simulink model "NumericalExampleWithSolids"  (R2024b)
settings: Solver=VariableStepDiscrete  StartTime=0.0  StopTime=T_final  MaxStep=0.4  MinStep=0.5  RelTol=1e-3
values from neighbouring files (symbols this model uses):
  loss_due_to_contamination = 0.3    [NumericalExampleWithSolids_param.m]
  m_ini_2_HDPE = 20    [NumericalExampleWithSolids_param.m]
  m_ini_2_PET = 20    [NumericalExampleWithSolids_param.m]
  m_ini_2_PP = 20    [NumericalExampleWithSolids_param.m]
  m_ini_3_HDPE = 100    [NumericalExampleWithSolids_param.m]
  m_ini_3_PET = 150    [NumericalExampleWithSolids_param.m]
  m_ini_3_PP = 120    [NumericalExampleWithSolids_param.m]
  m_ini_HDPE = 4.1    [NumericalExampleWithSolids_param.m]
  m_ini_PET = 8.1    [NumericalExampleWithSolids_param.m]
  m_ini_PP = 4.4    [NumericalExampleWithSolids_param.m]
  m_ini_Transport1to2_HDPE = 0    [NumericalExampleWithSolids_param.m]
  m_ini_Transport1to2_PET = 0    [NumericalExampleWithSolids_param.m]
  m_ini_Transport1to2_PP = 0    [NumericalExampleWithSolids_param.m]
  m_ini_Transport2to1_HDPE = 0    [NumericalExampleWithSolids_param.m]
  m_ini_Transport2to1_PET = 0    [NumericalExampleWithSolids_param.m]
  m_ini_Transport2to1_PP = 0    [NumericalExampleWithSolids_param.m]
  m_ini_Transport3to1_HDPE = 0    [NumericalExampleWithSolids_param.m]
  m_ini_Transport3to1_PET = 0    [NumericalExampleWithSolids_param.m]
  m_ini_Transport3to1_PP = 0    [NumericalExampleWithSolids_param.m]
  m_out_3_HDPE = 0.5    [NumericalExampleWithSolids_param.m]
  m_out_3_PET = 2    [NumericalExampleWithSolids_param.m]
  m_out_3_PP = 1    [NumericalExampleWithSolids_param.m]
  m_out_HDPE = 4.1    [NumericalExampleWithSolids_param.m]
  m_out_PET = 8.1    [NumericalExampleWithSolids_param.m]
  m_out_PP = 4.4    [NumericalExampleWithSolids_param.m]
  t_out_2_HDPE = t_out_Transport1to2_HDPE + recycling_time    (= 260)    [NumericalExampleWithSolids_param.m]
  t_out_2_PET = t_out_Transport1to2_PET + recycling_time    (= 260)    [NumericalExampleWithSolids_param.m]
  t_out_2_PP = t_out_Transport1to2_PP + recycling_time    (= 260)    [NumericalExampleWithSolids_param.m]
  t_out_3_HDPE = 1    [NumericalExampleWithSolids_param.m]
  t_out_3_PET = 1    [NumericalExampleWithSolids_param.m]
  t_out_3_PP = 1    [NumericalExampleWithSolids_param.m]
  t_out_HDPE = 100    [NumericalExampleWithSolids_param.m]
  t_out_PET = 100    [NumericalExampleWithSolids_param.m]
  t_out_PP = 100    [NumericalExampleWithSolids_param.m]
  t_out_Transport1to2_HDPE = t_out_HDPE + transportation_time_1to2    (= 220)    [NumericalExampleWithSolids_param.m]
  t_out_Transport1to2_PET = t_out_PET + transportation_time_1to2    (= 220)    [NumericalExampleWithSolids_param.m]
  t_out_Transport1to2_PP = t_out_PP + transportation_time_1to2    (= 220)    [NumericalExampleWithSolids_param.m]
  t_out_Transport2to1_HDPE = t_out_2_HDPE + transportation_time_2to1    (= 290)    [NumericalExampleWithSolids_param.m]
  t_out_Transport2to1_PET = t_out_2_PET + transportation_time_2to1    (= 290)    [NumericalExampleWithSolids_param.m]
  t_out_Transport2to1_PP = t_out_2_PP + transportation_time_2to1    (= 290)    [NumericalExampleWithSolids_param.m]
  t_out_Transport3to1_HDPE = t_out_3_HDPE + transportation_time_3to1    (= 7)    [NumericalExampleWithSolids_param.m]
  t_out_Transport3to1_PET = t_out_3_PET + transportation_time_3to1    (= 7)    [NumericalExampleWithSolids_param.m]
  t_out_Transport3to1_PP = t_out_3_PP + transportation_time_3to1    (= 7)    [NumericalExampleWithSolids_param.m]
  transportation_time_1to2 = 60*hours_for_transportation_1to2    (= 120)    [NumericalExampleWithSolids_param.m]
  transportation_time_2to1 = 60*hours_for_transportation_2to1    (= 30)    [NumericalExampleWithSolids_param.m]
  transportation_time_3to1 = 60*hours_for_transportation_3to1    (= 6)    [NumericalExampleWithSolids_param.m]
libraries: dspstat3 x1

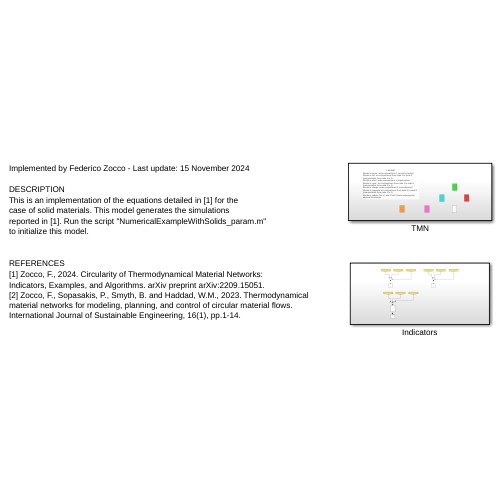
[thumbnail: Simulink's stored preview of the top-level diagram]
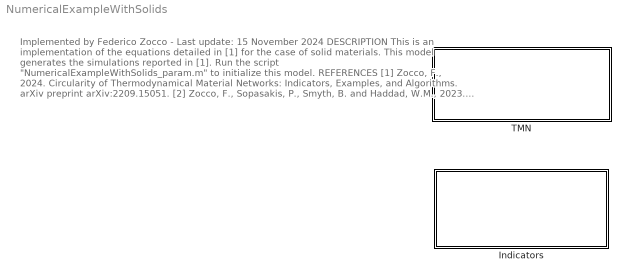
== system NumericalExampleWithSolids ==
  note: Implemented by Federico Zocco - Last update: 15 November 2024
      |
      | DESCRIPTION
      | This is an implementation of the equations detailed in [1] for the
      | case of solid materials. This model generates the simulations
      | reported in [1]. Run the script "NumericalExampleWithSolids_param.m"
      | to initialize this model.
      |
      | REFERENCES
      | [1] Zocco, F., 2024. Circularity of Thermodynamical Material Networks:
      | Indicators, Examples, and Algorithms. arXiv preprint arXiv:2209.15051.
      | [2] Zocco, F., Sopasakis, P., Smyth, B. and Haddad, W.M., 2023. Thermodynamical material networks for modeling, planning, and control of circular material flows. International Journal of Sustainable Engineering, 16(1), pp.1-14.
  Indicators : Subsystem
  TMN : Subsystem

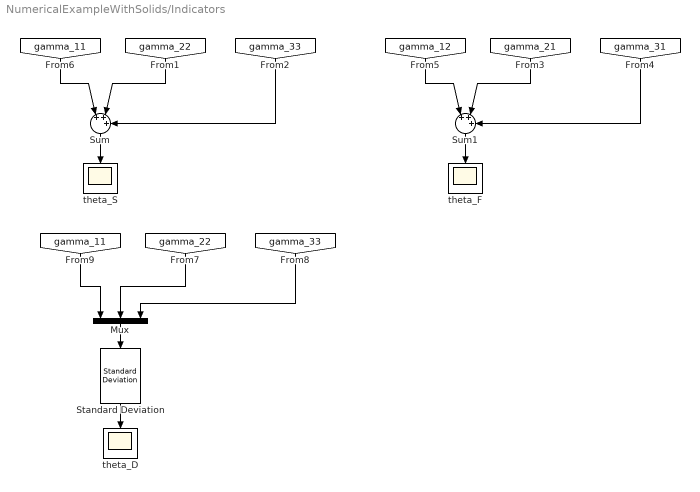
== system NumericalExampleWithSolids/Indicators ==
  Mux : Mux  Inputs=3
  Standard Deviation : dspstat3/Standard Deviation  run=off  directionMode=Each column  dimension=1  InputProcessing=Columns as channels (frame based)  reset_popup=None  roiEnable=off  roiType=Rectangles  roiPortion=Entire ROI  roiOutput=Individual statistics for each ROI  roiFlag=off
  Sum : Sum  Inputs=|+++
  Sum1 : Sum  Inputs=|+++
  theta_D : Scope
  theta_F : Scope
  theta_S : Scope
  wires:
  Mux/1 -> Standard Deviation/1
  [gamma_12] -> Sum1/1
  [gamma_22] -> Mux/2
  Sum/1 -> theta_S/1
  [gamma_33] -> Mux/3
  Standard Deviation/1 -> theta_D/1
  [gamma_11] -> Sum/1
  [gamma_33] -> Sum/3
  [gamma_31] -> Sum1/3
  Sum1/1 -> theta_F/1
  [gamma_21] -> Sum1/2
  [gamma_22] -> Sum/2
  [gamma_11] -> Mux/1

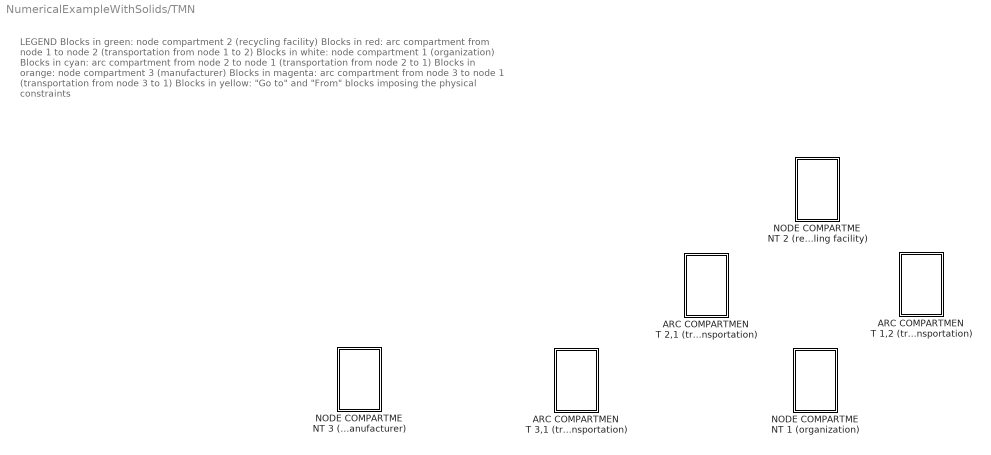
== system NumericalExampleWithSolids/TMN ==
  note: LEGEND
      | Blocks in green: node compartment 2 (recycling facility)
      | Blocks in red: arc compartment from node 1 to node 2 (transportation from node 1 to 2)
      | Blocks in white: node compartment 1 (organization)
      | Blocks in cyan: arc compartment from node 2 to node 1 (transportation from node 2 to 1)
      | Blocks in orange: node compartment 3 (manufacturer)
      | Blocks in magenta: arc compartment from node 3 to node 1 (transportation from node 3 to 1)
      | Blocks in yellow: "Go to" and "From" blocks imposing the physical constraints
  ARC COMPARTMENT 1,2 (transportation) : Subsystem
  ARC COMPARTMENT 2,1 (transportation) : Subsystem
  ARC COMPARTMENT 3,1 (transportation) : Subsystem
  NODE COMPARTMENT 1 (organization) : Subsystem
  NODE COMPARTMENT 2 (recycling facility) : Subsystem
  NODE COMPARTMENT 3 (manufacturer) : Subsystem

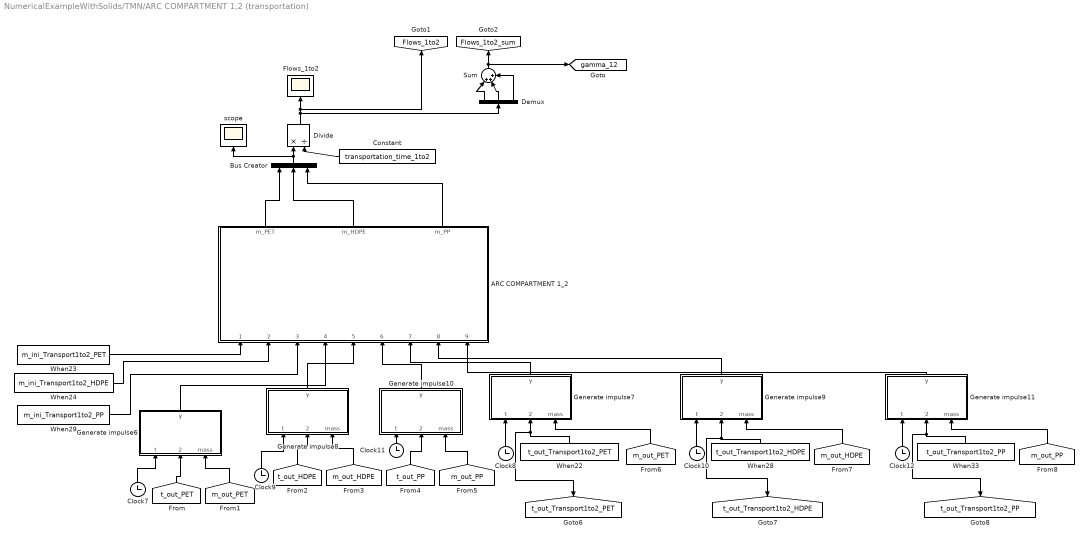
== system NumericalExampleWithSolids/TMN/ARC COMPARTMENT 1,2 (transportation) ==
  ARC COMPARTMENT 1_2 : MATLAB Function  TreatAsAtomicUnit=on
  Bus Creator : BusCreator  Inputs=3
  Clock{7..12} (6 alike) : Clock
  Constant : Constant  Value=transportation_time_1to2
  Demux : Demux  Outputs=3
  Divide : Product  Inputs=*/
  Flows_1to2 : Scope
  Generate impulse10 : MATLAB Function  TreatAsAtomicUnit=on
  Generate impulse11 : MATLAB Function  TreatAsAtomicUnit=on
  Generate impulse6 : MATLAB Function  TreatAsAtomicUnit=on
  Generate impulse7 : MATLAB Function  TreatAsAtomicUnit=on
  Generate impulse8 : MATLAB Function  TreatAsAtomicUnit=on
  Generate impulse9 : MATLAB Function  TreatAsAtomicUnit=on
  Sum : Sum  Inputs=|+++
  When22 : Constant  Value=t_out_Transport1to2_PET
  When23 : Constant  Value=m_ini_Transport1to2_PET
  When24 : Constant  Value=m_ini_Transport1to2_HDPE
  When28 : Constant  Value=t_out_Transport1to2_HDPE
  When29 : Constant  Value=m_ini_Transport1to2_PP
  When33 : Constant  Value=t_out_Transport1to2_PP
  scope : Scope
  tag scope: Flows_1to2=global, Flows_1to2_sum=global, gamma_12=global, t_out_Transport1to2_HDPE=global, t_out_Transport1to2_PET=global, t_out_Transport1to2_PP=global
  wires:
  Generate impulse6/1(y) -> ARC COMPARTMENT 1_2/4(m_in_Transport1to2_PET)
  [m_out_PET] -> Generate impulse7/3(mass)
  Generate impulse11/1(y) -> ARC COMPARTMENT 1_2/9(m_out_Transport1to2_PP)
  ARC COMPARTMENT 1_2/3(m_PP) -> Bus Creator/3
  Bus Creator/1 -> scope/1, Divide/1
  [m_out_PP] -> Generate impulse10/3(mass)
  Clock7/1 -> Generate impulse6/1(t)
  Generate impulse10/1(y) -> ARC COMPARTMENT 1_2/6(m_in_Transport1to2_PP)
  Generate impulse9/1(y) -> ARC COMPARTMENT 1_2/8(m_out_Transport1to2_HDPE)
  [m_out_PET] -> Generate impulse6/3(mass)
  [t_out_HDPE] -> Generate impulse8/2(n_impulse)
  Generate impulse7/1(y) -> ARC COMPARTMENT 1_2/7(m_out_Transport1to2_PET)
  Constant/1 -> Divide/2
  When28/1 -> [t_out_Transport1to2_HDPE], Generate impulse9/2(n_impulse)
  Clock10/1 -> Generate impulse9/1(t)
  When29/1 -> ARC COMPARTMENT 1_2/3(m_ini_Transport1to2_PP)
  When22/1 -> [t_out_Transport1to2_PET], Generate impulse7/2(n_impulse)
  Clock8/1 -> Generate impulse7/1(t)
  Generate impulse8/1(y) -> ARC COMPARTMENT 1_2/5(m_in_Transport1to2_HDPE)
  When23/1 -> ARC COMPARTMENT 1_2/1(m_ini_Transport1to2_PET)
  ARC COMPARTMENT 1_2/2(m_HDPE) -> Bus Creator/2
  [m_out_HDPE] -> Generate impulse9/3(mass)
  Clock9/1 -> Generate impulse8/1(t)
  When24/1 -> ARC COMPARTMENT 1_2/2(m_ini_Transport1to2_HDPE)
  ARC COMPARTMENT 1_2/1(m_PET) -> Bus Creator/1
  Clock11/1 -> Generate impulse10/1(t)
  [t_out_PET] -> Generate impulse6/2(n_impulse)
  [t_out_PP] -> Generate impulse10/2(n_impulse)
  Clock12/1 -> Generate impulse11/1(t)
  [m_out_HDPE] -> Generate impulse8/3(mass)
  When33/1 -> [t_out_Transport1to2_PP], Generate impulse11/2(n_impulse)
  [m_out_PP] -> Generate impulse11/3(mass)
  Demux/1 -> Sum/1
  Demux/3 -> Sum/3
  Divide/1 -> Demux/1, [Flows_1to2], Flows_1to2/1
  Demux/2 -> Sum/2
  Sum/1 -> [Flows_1to2_sum], [gamma_12]

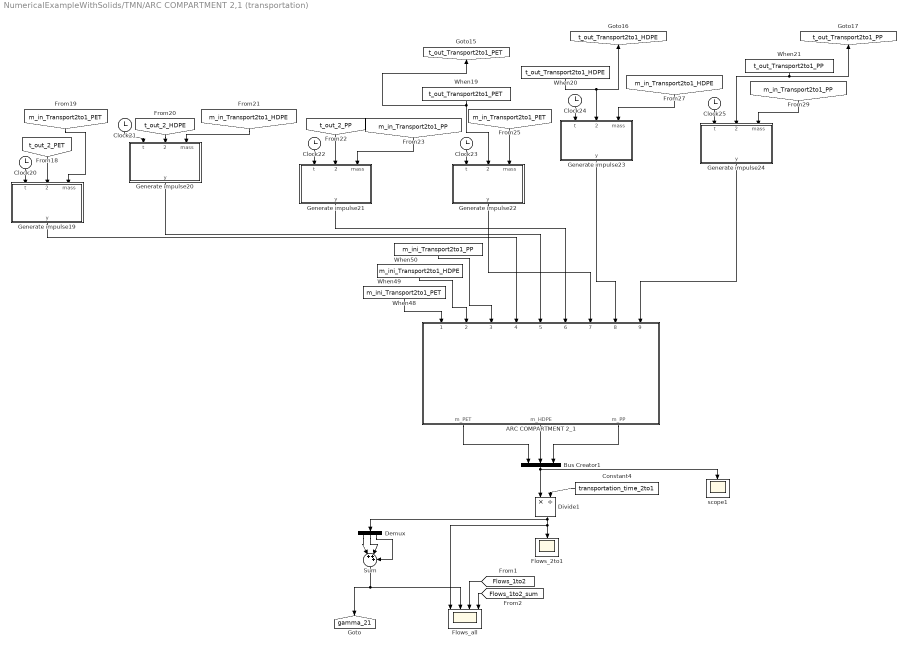
== system NumericalExampleWithSolids/TMN/ARC COMPARTMENT 2,1 (transportation) ==
  ARC COMPARTMENT 2_1 : MATLAB Function  TreatAsAtomicUnit=on
  Bus Creator1 : BusCreator  Inputs=3
  Clock{20..25} (6 alike) : Clock
  Constant4 : Constant  Value=transportation_time_2to1
  Demux : Demux  Outputs=3
  Divide1 : Product  Inputs=*/
  Flows_2to1 : Scope
  Flows_all : Scope  NumInputPorts=4
  Generate impulse19 : MATLAB Function  TreatAsAtomicUnit=on
  Generate impulse20 : MATLAB Function  TreatAsAtomicUnit=on
  Generate impulse21 : MATLAB Function  TreatAsAtomicUnit=on
  Generate impulse22 : MATLAB Function  TreatAsAtomicUnit=on
  Generate impulse23 : MATLAB Function  TreatAsAtomicUnit=on
  Generate impulse24 : MATLAB Function  TreatAsAtomicUnit=on
  Sum : Sum  Inputs=|+++
  When19 : Constant  Value=t_out_Transport2to1_PET
  When20 : Constant  Value=t_out_Transport2to1_HDPE
  When21 : Constant  Value=t_out_Transport2to1_PP
  When48 : Constant  Value=m_ini_Transport2to1_PET
  When49 : Constant  Value=m_ini_Transport2to1_HDPE
  When50 : Constant  Value=m_ini_Transport2to1_PP
  scope1 : Scope
  tag scope: gamma_21=global, t_out_Transport2to1_HDPE=global, t_out_Transport2to1_PET=global, t_out_Transport2to1_PP=global
  wires:
  [m_in_Transport2to1_PP] -> Generate impulse24/3(mass)
  ARC COMPARTMENT 2_1/2(m_HDPE) -> Bus Creator1/2
  Clock23/1 -> Generate impulse22/1(t)
  Generate impulse20/1(y) -> ARC COMPARTMENT 2_1/5(m_in_Transport2to1_HDPE)
  When49/1 -> ARC COMPARTMENT 2_1/2(m_ini_Transport2to1_HDPE)
  Clock21/1 -> Generate impulse20/1(t)
  Generate impulse21/1(y) -> ARC COMPARTMENT 2_1/6(m_in_Transport2to1_PP)
  Clock20/1 -> Generate impulse19/1(t)
  [m_in_Transport2to1_HDPE] -> Generate impulse23/3(mass)
  When21/1 -> Generate impulse24/2(n_impulse), [t_out_Transport2to1_PP]
  When48/1 -> ARC COMPARTMENT 2_1/1(m_ini_Transport2to1_PET)
  When20/1 -> [t_out_Transport2to1_HDPE], Generate impulse23/2(n_impulse)
  Generate impulse19/1(y) -> ARC COMPARTMENT 2_1/4(m_in_Transport2to1_PET)
  ARC COMPARTMENT 2_1/1(m_PET) -> Bus Creator1/1
  [m_in_Transport2to1_PP] -> Generate impulse21/3(mass)
  [m_in_Transport2to1_HDPE] -> Generate impulse20/3(mass)
  Clock22/1 -> Generate impulse21/1(t)
  When19/1 -> [t_out_Transport2to1_PET], Generate impulse22/2(n_impulse)
  [t_out_2_PET] -> Generate impulse19/2(n_impulse)
  Bus Creator1/1 -> Divide1/1, scope1/1
  Clock25/1 -> Generate impulse24/1(t)
  When50/1 -> ARC COMPARTMENT 2_1/3(m_ini_Transport2to1_PP)
  [t_out_2_PP] -> Generate impulse21/2(n_impulse)
  Divide1/1 -> Demux/1, Flows_all/1, Flows_2to1/1
  [m_in_Transport2to1_PET] -> Generate impulse19/3(mass)
  [t_out_2_HDPE] -> Generate impulse20/2(n_impulse)
  Generate impulse24/1(y) -> ARC COMPARTMENT 2_1/9(m_out_Transport2to1_PP)
  Clock24/1 -> Generate impulse23/1(t)
  [m_in_Transport2to1_PET] -> Generate impulse22/3(mass)
  ARC COMPARTMENT 2_1/3(m_PP) -> Bus Creator1/3
  Constant4/1 -> Divide1/2
  Generate impulse23/1(y) -> ARC COMPARTMENT 2_1/8(m_out_Transport2to1_HDPE)
  Generate impulse22/1(y) -> ARC COMPARTMENT 2_1/7(m_out_Transport2to1_PET)
  [Flows_1to2] -> Flows_all/3
  Sum/1 -> Flows_all/2, [gamma_21]
  Demux/1 -> Sum/1
  Demux/2 -> Sum/2
  Demux/3 -> Sum/3
  [Flows_1to2_sum] -> Flows_all/4

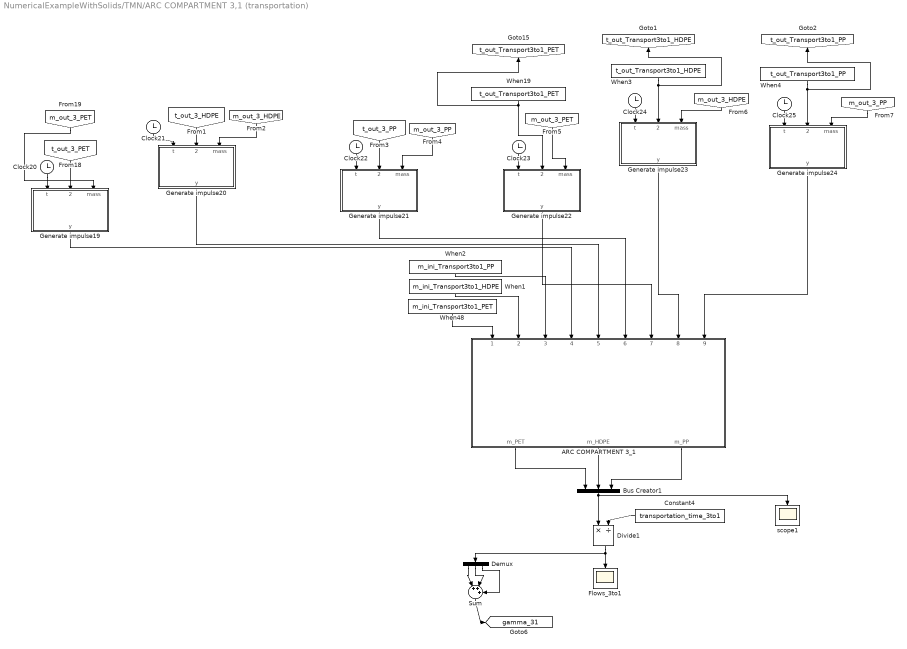
== system NumericalExampleWithSolids/TMN/ARC COMPARTMENT 3,1 (transportation) ==
  ARC COMPARTMENT 3_1 : MATLAB Function  TreatAsAtomicUnit=on
  Bus Creator1 : BusCreator  Inputs=3
  Clock{20..25} (6 alike) : Clock
  Constant4 : Constant  Value=transportation_time_3to1
  Demux : Demux  Outputs=3
  Divide1 : Product  Inputs=*/
  Flows_3to1 : Scope
  Generate impulse19 : MATLAB Function  TreatAsAtomicUnit=on
  Generate impulse20 : MATLAB Function  TreatAsAtomicUnit=on
  Generate impulse21 : MATLAB Function  TreatAsAtomicUnit=on
  Generate impulse22 : MATLAB Function  TreatAsAtomicUnit=on
  Generate impulse23 : MATLAB Function  TreatAsAtomicUnit=on
  Generate impulse24 : MATLAB Function  TreatAsAtomicUnit=on
  Sum : Sum  Inputs=|+++
  When1 : Constant  Value=m_ini_Transport3to1_HDPE
  When19 : Constant  Value=t_out_Transport3to1_PET
  When2 : Constant  Value=m_ini_Transport3to1_PP
  When3 : Constant  Value=t_out_Transport3to1_HDPE
  When4 : Constant  Value=t_out_Transport3to1_PP
  When48 : Constant  Value=m_ini_Transport3to1_PET
  scope1 : Scope
  tag scope: gamma_31=global, t_out_Transport3to1_HDPE=global, t_out_Transport3to1_PET=global, t_out_Transport3to1_PP=global
  wires:
  [m_out_3_PP] -> Generate impulse24/3(mass)
  ARC COMPARTMENT 3_1/2(m_HDPE) -> Bus Creator1/2
  Clock23/1 -> Generate impulse22/1(t)
  Generate impulse20/1(y) -> ARC COMPARTMENT 3_1/5(m_in_Transport3to1_HDPE)
  When1/1 -> ARC COMPARTMENT 3_1/2(m_ini_Transport3to1_HDPE)
  Clock21/1 -> Generate impulse20/1(t)
  Generate impulse21/1(y) -> ARC COMPARTMENT 3_1/6(m_in_Transport3to1_PP)
  Clock20/1 -> Generate impulse19/1(t)
  [m_out_3_HDPE] -> Generate impulse23/3(mass)
  When4/1 -> Generate impulse24/2(n_impulse), [t_out_Transport3to1_PP]
  When48/1 -> ARC COMPARTMENT 3_1/1(m_ini_Transport3to1_PET)
  Generate impulse19/1(y) -> ARC COMPARTMENT 3_1/4(m_in_Transport3to1_PET)
  ARC COMPARTMENT 3_1/1(m_PET) -> Bus Creator1/1
  [m_out_3_PP] -> Generate impulse21/3(mass)
  [m_out_3_HDPE] -> Generate impulse20/3(mass)
  Clock22/1 -> Generate impulse21/1(t)
  When19/1 -> [t_out_Transport3to1_PET], Generate impulse22/2(n_impulse)
  [t_out_3_PET] -> Generate impulse19/2(n_impulse)
  Bus Creator1/1 -> Divide1/1, scope1/1
  Clock25/1 -> Generate impulse24/1(t)
  When2/1 -> ARC COMPARTMENT 3_1/3(m_ini_Transport3to1_PP)
  [t_out_3_PP] -> Generate impulse21/2(n_impulse)
  [m_out_3_PET] -> Generate impulse19/3(mass)
  [t_out_3_HDPE] -> Generate impulse20/2(n_impulse)
  Generate impulse24/1(y) -> ARC COMPARTMENT 3_1/9(m_out_Transport3to1_PP)
  Clock24/1 -> Generate impulse23/1(t)
  [m_out_3_PET] -> Generate impulse22/3(mass)
  ARC COMPARTMENT 3_1/3(m_PP) -> Bus Creator1/3
  Constant4/1 -> Divide1/2
  Generate impulse23/1(y) -> ARC COMPARTMENT 3_1/8(m_out_Transport3to1_HDPE)
  Generate impulse22/1(y) -> ARC COMPARTMENT 3_1/7(m_out_Transport3to1_PET)
  When3/1 -> Generate impulse23/2(n_impulse), [t_out_Transport3to1_HDPE]
  Demux/2 -> Sum/2
  Sum/1 -> [gamma_31]
  Demux/1 -> Sum/1
  Divide1/1 -> Demux/1, Flows_3to1/1
  Demux/3 -> Sum/3

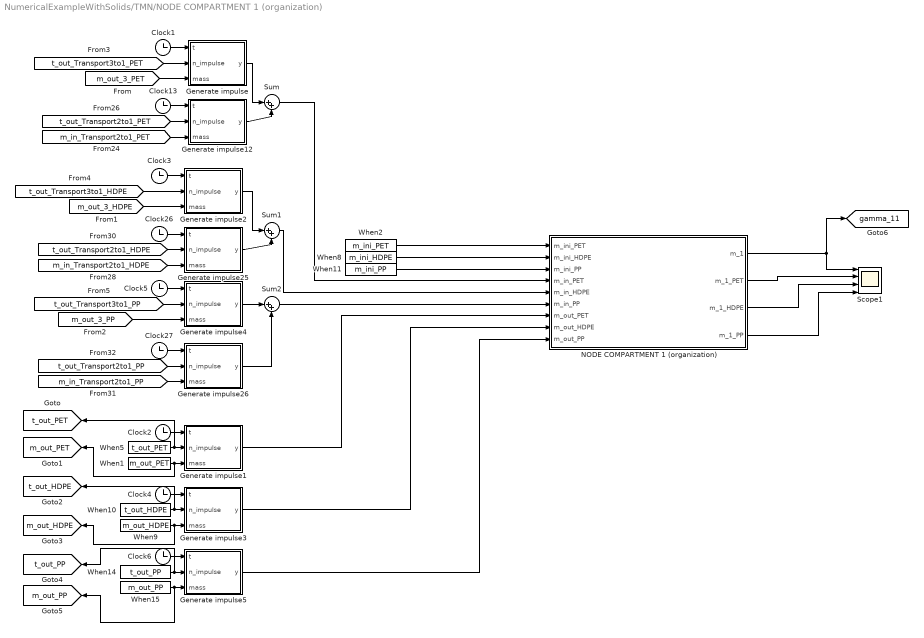
== system NumericalExampleWithSolids/TMN/NODE COMPARTMENT 1 (organization) ==
  Clock{1..6,13,26..27} (9 alike) : Clock
  Generate impulse : MATLAB Function  TreatAsAtomicUnit=on
  Generate impulse1 : MATLAB Function  TreatAsAtomicUnit=on
  Generate impulse12 : MATLAB Function  TreatAsAtomicUnit=on
  Generate impulse2 : MATLAB Function  TreatAsAtomicUnit=on
  Generate impulse25 : MATLAB Function  TreatAsAtomicUnit=on
  Generate impulse26 : MATLAB Function  TreatAsAtomicUnit=on
  Generate impulse3 : MATLAB Function  TreatAsAtomicUnit=on
  Generate impulse4 : MATLAB Function  TreatAsAtomicUnit=on
  Generate impulse5 : MATLAB Function  TreatAsAtomicUnit=on
  NODE COMPARTMENT 1 (organization) : MATLAB Function  TreatAsAtomicUnit=on
  Scope1 : Scope  NumInputPorts=4
  Sum : Sum  Inputs=|++
  Sum1 : Sum  Inputs=|++
  Sum2 : Sum  Inputs=|++
  When1 : Constant  Value=m_out_PET
  When10 : Constant  Value=t_out_HDPE
  When11 : Constant  Value=m_ini_PP
  When14 : Constant  Value=t_out_PP
  When15 : Constant  Value=m_out_PP
  When2 : Constant  Value=m_ini_PET
  When5 : Constant  Value=t_out_PET
  When8 : Constant  Value=m_ini_HDPE
  When9 : Constant  Value=m_out_HDPE
  tag scope: gamma_11=global, m_out_HDPE=global, m_out_PET=global, m_out_PP=global, t_out_HDPE=global, t_out_PET=global, t_out_PP=global
  wires:
  [m_out_3_HDPE] -> Generate impulse2/3(mass)
  Sum1/1 -> NODE COMPARTMENT 1 (organization)/5(m_in_HDPE)
  [t_out_Transport3to1_PP] -> Generate impulse4/2(n_impulse)
  [t_out_Transport3to1_HDPE] -> Generate impulse2/2(n_impulse)
  [m_in_Transport2to1_HDPE] -> Generate impulse25/3(mass)
  Clock2/1 -> Generate impulse1/1(t)
  Clock5/1 -> Generate impulse4/1(t)
  When2/1 -> NODE COMPARTMENT 1 (organization)/1(m_ini_PET)
  Clock3/1 -> Generate impulse2/1(t)
  Sum2/1 -> NODE COMPARTMENT 1 (organization)/6(m_in_PP)
  [m_out_3_PP] -> Generate impulse4/3(mass)
  Generate impulse1/1(y) -> NODE COMPARTMENT 1 (organization)/7(m_out_PET)
  Generate impulse/1(y) -> Sum/1
  NODE COMPARTMENT 1 (organization)/1(m_1) -> Scope1/1, [gamma_11]
  Generate impulse3/1(y) -> NODE COMPARTMENT 1 (organization)/8(m_out_HDPE)
  [t_out_Transport2to1_PP] -> Generate impulse26/2(n_impulse)
  Clock27/1 -> Generate impulse26/1(t)
  Clock4/1 -> Generate impulse3/1(t)
  When10/1 -> [t_out_HDPE], Generate impulse3/2(n_impulse)
  Clock26/1 -> Generate impulse25/1(t)
  When11/1 -> NODE COMPARTMENT 1 (organization)/3(m_ini_PP)
  [m_in_Transport2to1_PET] -> Generate impulse12/3(mass)
  [t_out_Transport2to1_HDPE] -> Generate impulse25/2(n_impulse)
  Generate impulse25/1(y) -> Sum1/2
  Clock13/1 -> Generate impulse12/1(t)
  When15/1 -> [m_out_PP], Generate impulse5/3(mass)
  [m_in_Transport2to1_PP] -> Generate impulse26/3(mass)
  Generate impulse4/1(y) -> Sum2/1
  Generate impulse26/1(y) -> Sum2/2
  Clock1/1 -> Generate impulse/1(t)
  When14/1 -> [t_out_PP], Generate impulse5/2(n_impulse)
  When5/1 -> [t_out_PET], Generate impulse1/2(n_impulse)
  When8/1 -> NODE COMPARTMENT 1 (organization)/2(m_ini_HDPE)
  [t_out_Transport2to1_PET] -> Generate impulse12/2(n_impulse)
  Generate impulse12/1(y) -> Sum/2
  Generate impulse5/1(y) -> NODE COMPARTMENT 1 (organization)/9(m_out_PP)
  When9/1 -> [m_out_HDPE], Generate impulse3/3(mass)
  Clock6/1 -> Generate impulse5/1(t)
  NODE COMPARTMENT 1 (organization)/4(m_1_PP) -> Scope1/4
  When1/1 -> [m_out_PET], Generate impulse1/3(mass)
  NODE COMPARTMENT 1 (organization)/3(m_1_HDPE) -> Scope1/3
  NODE COMPARTMENT 1 (organization)/2(m_1_PET) -> Scope1/2
  Generate impulse2/1(y) -> Sum1/1
  [m_out_3_PET] -> Generate impulse/3(mass)
  Sum/1 -> NODE COMPARTMENT 1 (organization)/4(m_in_PET)
  [t_out_Transport3to1_PET] -> Generate impulse/2(n_impulse)

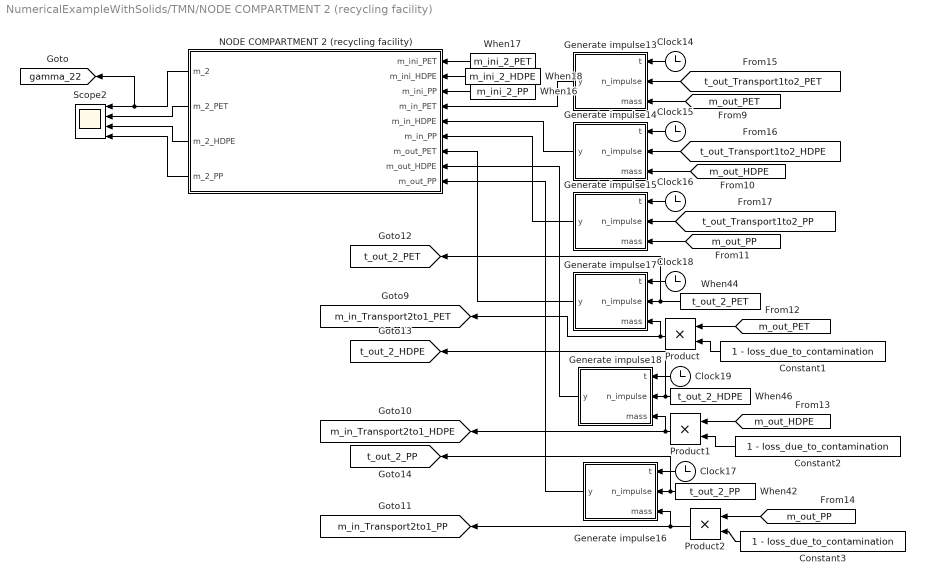
== system NumericalExampleWithSolids/TMN/NODE COMPARTMENT 2 (recycling facility) ==
  Clock{14..19} (6 alike) : Clock
  Constant1 : Constant  Value=1 - loss_due_to_contamination
  Constant2 : Constant  Value=1 - loss_due_to_contamination
  Constant3 : Constant  Value=1 - loss_due_to_contamination
  Generate impulse13 : MATLAB Function  TreatAsAtomicUnit=on
  Generate impulse14 : MATLAB Function  TreatAsAtomicUnit=on
  Generate impulse15 : MATLAB Function  TreatAsAtomicUnit=on
  Generate impulse16 : MATLAB Function  TreatAsAtomicUnit=on
  Generate impulse17 : MATLAB Function  TreatAsAtomicUnit=on
  Generate impulse18 : MATLAB Function  TreatAsAtomicUnit=on
  NODE COMPARTMENT 2 (recycling facility) : MATLAB Function  TreatAsAtomicUnit=on
  Product : Product
  Product1 : Product
  Product2 : Product
  Scope2 : Scope  NumInputPorts=4
  When16 : Constant  Value=m_ini_2_PP
  When17 : Constant  Value=m_ini_2_PET
  When18 : Constant  Value=m_ini_2_HDPE
  When42 : Constant  Value=t_out_2_PP
  When44 : Constant  Value=t_out_2_PET
  When46 : Constant  Value=t_out_2_HDPE
  tag scope: gamma_22=global, m_in_Transport2to1_HDPE=global, m_in_Transport2to1_PET=global, m_in_Transport2to1_PP=global, t_out_2_HDPE=global, t_out_2_PET=global, t_out_2_PP=global
  wires:
  NODE COMPARTMENT 2 (recycling facility)/2(m_2_PET) -> Scope2/2
  NODE COMPARTMENT 2 (recycling facility)/3(m_2_HDPE) -> Scope2/3
  NODE COMPARTMENT 2 (recycling facility)/4(m_2_PP) -> Scope2/4
  Constant3/1 -> Product2/2
  [t_out_Transport1to2_PP] -> Generate impulse15/2(n_impulse)
  Generate impulse15/1(y) -> NODE COMPARTMENT 2 (recycling facility)/6(m_in_PP)
  [m_out_PP] -> Product2/1
  Product2/1 -> Generate impulse16/3(mass), [m_in_Transport2to1_PP]
  Clock19/1 -> Generate impulse18/1(t)
  Generate impulse16/1(y) -> NODE COMPARTMENT 2 (recycling facility)/9(m_out_PP)
  Generate impulse18/1(y) -> NODE COMPARTMENT 2 (recycling facility)/8(m_out_HDPE)
  When42/1 -> [t_out_2_PP], Generate impulse16/2(n_impulse)
  When16/1 -> NODE COMPARTMENT 2 (recycling facility)/3(m_ini_PP)
  [t_out_Transport1to2_HDPE] -> Generate impulse14/2(n_impulse)
  Product1/1 -> Generate impulse18/3(mass), [m_in_Transport2to1_HDPE]
  When18/1 -> NODE COMPARTMENT 2 (recycling facility)/2(m_ini_HDPE)
  [m_out_PP] -> Generate impulse15/3(mass)
  Clock18/1 -> Generate impulse17/1(t)
  [t_out_Transport1to2_PET] -> Generate impulse13/2(n_impulse)
  Clock16/1 -> Generate impulse15/1(t)
  Generate impulse14/1(y) -> NODE COMPARTMENT 2 (recycling facility)/5(m_in_HDPE)
  When17/1 -> NODE COMPARTMENT 2 (recycling facility)/1(m_ini_PET)
  Product/1 -> [m_in_Transport2to1_PET], Generate impulse17/3(mass)
  Clock15/1 -> Generate impulse14/1(t)
  Constant1/1 -> Product/2
  NODE COMPARTMENT 2 (recycling facility)/1(m_2) -> [gamma_22], Scope2/1
  Generate impulse13/1(y) -> NODE COMPARTMENT 2 (recycling facility)/4(m_in_PET)
  [m_out_PET] -> Product/1
  [m_out_HDPE] -> Generate impulse14/3(mass)
  [m_out_HDPE] -> Product1/1
  Clock17/1 -> Generate impulse16/1(t)
  When44/1 -> [t_out_2_PET], Generate impulse17/2(n_impulse)
  [m_out_PET] -> Generate impulse13/3(mass)
  Clock14/1 -> Generate impulse13/1(t)
  Constant2/1 -> Product1/2
  When46/1 -> [t_out_2_HDPE], Generate impulse18/2(n_impulse)
  Generate impulse17/1(y) -> NODE COMPARTMENT 2 (recycling facility)/7(m_out_PET)

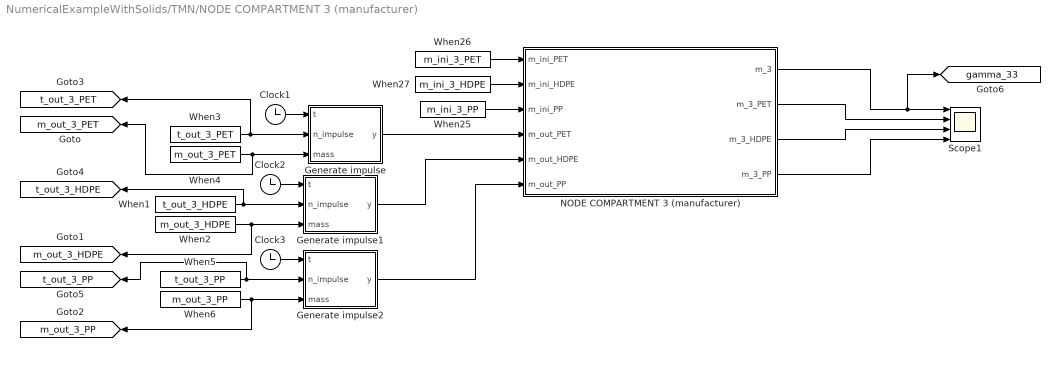
== system NumericalExampleWithSolids/TMN/NODE COMPARTMENT 3 (manufacturer) ==
  Clock1 : Clock
  Clock2 : Clock
  Clock3 : Clock
  Generate impulse : MATLAB Function  TreatAsAtomicUnit=on
  Generate impulse1 : MATLAB Function  TreatAsAtomicUnit=on
  Generate impulse2 : MATLAB Function  TreatAsAtomicUnit=on
  NODE COMPARTMENT 3 (manufacturer) : MATLAB Function  TreatAsAtomicUnit=on
  Scope1 : Scope  NumInputPorts=4
  When1 : Constant  Value=t_out_3_HDPE
  When2 : Constant  Value=m_out_3_HDPE
  When25 : Constant  Value=m_ini_3_PP
  When26 : Constant  Value=m_ini_3_PET
  When27 : Constant  Value=m_ini_3_HDPE
  When3 : Constant  Value=t_out_3_PET
  When4 : Constant  Value=m_out_3_PET
  When5 : Constant  Value=t_out_3_PP
  When6 : Constant  Value=m_out_3_PP
  tag scope: gamma_33=global, m_out_3_HDPE=global, m_out_3_PET=global, m_out_3_PP=global, t_out_3_HDPE=global, t_out_3_PET=global, t_out_3_PP=global
  wires:
  NODE COMPARTMENT 3 (manufacturer)/2(m_3_PET) -> Scope1/2
  Generate impulse1/1(y) -> NODE COMPARTMENT 3 (manufacturer)/5(m_out_HDPE)
  Generate impulse/1(y) -> NODE COMPARTMENT 3 (manufacturer)/4(m_out_PET)
  When1/1 -> Generate impulse1/2(n_impulse), [t_out_3_HDPE]
  When3/1 -> [t_out_3_PET], Generate impulse/2(n_impulse)
  Generate impulse2/1(y) -> NODE COMPARTMENT 3 (manufacturer)/6(m_out_PP)
  When27/1 -> NODE COMPARTMENT 3 (manufacturer)/2(m_ini_HDPE)
  When25/1 -> NODE COMPARTMENT 3 (manufacturer)/3(m_ini_PP)
  NODE COMPARTMENT 3 (manufacturer)/3(m_3_HDPE) -> Scope1/3
  Clock3/1 -> Generate impulse2/1(t)
  NODE COMPARTMENT 3 (manufacturer)/1(m_3) -> [gamma_33], Scope1/1
  When6/1 -> [m_out_3_PP], Generate impulse2/3(mass)
  NODE COMPARTMENT 3 (manufacturer)/4(m_3_PP) -> Scope1/4
  When5/1 -> [t_out_3_PP], Generate impulse2/2(n_impulse)
  When2/1 -> [m_out_3_HDPE], Generate impulse1/3(mass)
  When26/1 -> NODE COMPARTMENT 3 (manufacturer)/1(m_ini_PET)
  Clock2/1 -> Generate impulse1/1(t)
  Clock1/1 -> Generate impulse/1(t)
  When4/1 -> [m_out_3_PET], Generate impulse/3(mass)

== matlab function NumericalExampleWithSolids/TMN/ARC COMPARTMENT 1,2 (transportation)/Generate impulse6 ==
  data: t input; y output; n_impulse input; mass input
function y = fcn(t, n_impulse, mass)

rectangleWidthToMakeImpulse = 0.4;

y = mass*rectpuls(t-n_impulse,rectangleWidthToMakeImpulse);

== matlab function NumericalExampleWithSolids/TMN/ARC COMPARTMENT 1,2 (transportation)/ARC COMPARTMENT 1_2 ==
  settings: updateMethod=DISCRETE
  data: m_ini_Transport1to2_PET input; m_ini_Transport1to2_HDPE input; m_ini_Transport1to2_PP input; m_in_Transport1to2_PET input; m_in_Transport1to2_HDPE input; m_in_Transport1to2_PP input; m_out_Transport1to2_PET input; m_PET output; m_out_Transport1to2_HDPE input; m_HDPE output; m_PP output; m_out_Transport1to2_PP input
function [m_PET, m_HDPE, m_PP] = fcn(m_ini_Transport1to2_PET, m_ini_Transport1to2_HDPE, m_ini_Transport1to2_PP, m_in_Transport1to2_PET, m_in_Transport1to2_HDPE, m_in_Transport1to2_PP, m_out_Transport1to2_PET, m_out_Transport1to2_HDPE, m_out_Transport1to2_PP)

persistent m_stock_PET;
persistent m_stock_HDPE;
persistent m_stock_PP;

if isempty(m_stock_PET) % t = 0
    m_stock_PET = m_ini_Transport1to2_PET;
    m_stock_HDPE = m_ini_Transport1to2_HDPE; 
    m_stock_PP = m_ini_Transport1to2_PP;
end

m_stock_PET = m_stock_PET + m_in_Transport1to2_PET - m_out_Transport1to2_PET;
m_stock_HDPE = m_stock_HDPE + m_in_Transport1to2_HDPE - m_out_Transport1to2_HDPE;
m_stock_PP = m_stock_PP + m_in_Transport1to2_PP - m_out_Transport1to2_PP;  

m_PET = m_stock_PET;
m_HDPE = m_stock_HDPE;
m_PP = m_stock_PP;

== matlab function NumericalExampleWithSolids/TMN/ARC COMPARTMENT 1,2 (transportation)/Generate impulse7 ==
  data: t input; y output; n_impulse input; mass input
function y = fcn(t, n_impulse, mass)

rectangleWidthToMakeImpulse = 0.4;

y = mass*rectpuls(t-n_impulse,rectangleWidthToMakeImpulse);

== matlab function NumericalExampleWithSolids/TMN/ARC COMPARTMENT 1,2 (transportation)/Generate impulse8 ==
  data: t input; y output; n_impulse input; mass input
function y = fcn(t, n_impulse, mass)

rectangleWidthToMakeImpulse = 0.4;

y = mass*rectpuls(t-n_impulse,rectangleWidthToMakeImpulse);

== matlab function NumericalExampleWithSolids/TMN/ARC COMPARTMENT 1,2 (transportation)/Generate impulse10 ==
  data: t input; y output; n_impulse input; mass input
function y = fcn(t, n_impulse, mass)

rectangleWidthToMakeImpulse = 0.4;

y = mass*rectpuls(t-n_impulse,rectangleWidthToMakeImpulse);

== matlab function NumericalExampleWithSolids/TMN/ARC COMPARTMENT 1,2 (transportation)/Generate impulse9 ==
  data: t input; y output; n_impulse input; mass input
function y = fcn(t, n_impulse, mass)

rectangleWidthToMakeImpulse = 0.4;

y = mass*rectpuls(t-n_impulse,rectangleWidthToMakeImpulse);

== matlab function NumericalExampleWithSolids/TMN/ARC COMPARTMENT 1,2 (transportation)/Generate impulse11 ==
  data: t input; y output; n_impulse input; mass input
function y = fcn(t, n_impulse, mass)

rectangleWidthToMakeImpulse = 0.4;

y = mass*rectpuls(t-n_impulse,rectangleWidthToMakeImpulse);

== matlab function NumericalExampleWithSolids/TMN/NODE COMPARTMENT 1 (organization)/Generate impulse12 ==
  data: t input; y output; n_impulse input; mass input
function y = fcn(t, n_impulse, mass)

rectangleWidthToMakeImpulse = 0.4; % epsilon

y = mass*rectpuls(t-n_impulse,rectangleWidthToMakeImpulse);

== matlab function NumericalExampleWithSolids/TMN/NODE COMPARTMENT 2 (recycling facility)/NODE COMPARTMENT 2 (recycling facility) ==
  settings: updateMethod=DISCRETE
  data: m_ini_PET input; m_ini_HDPE input; m_ini_PP input; m_in_PET input; m_in_HDPE input; m_in_PP input; m_2 output; m_out_PET input; m_out_HDPE input; m_out_PP input; m_2_PET output; m_2_HDPE output; m_2_PP output
function [m_2, m_2_PET, m_2_HDPE, m_2_PP] = fcn(m_ini_PET, m_ini_HDPE, m_ini_PP, m_in_PET, m_in_HDPE, m_in_PP, m_out_PET, m_out_HDPE, m_out_PP)

persistent m_stock;
persistent m_stock_PET;
persistent m_stock_HDPE;
persistent m_stock_PP;

if isempty(m_stock) % t = 0
    m_stock = m_ini_PET + m_ini_HDPE + m_ini_PP;
    m_stock_PET = m_ini_PET;
    m_stock_HDPE = m_ini_HDPE;
    m_stock_PP = m_ini_PP; 
end

m_stock = m_stock + m_in_PET + m_in_HDPE + m_in_PP - m_out_PET - m_out_HDPE - m_out_PP;
m_stock_PET = m_stock_PET + m_in_PET - m_out_PET;
m_stock_HDPE = m_stock_HDPE + m_in_HDPE - m_out_HDPE;
m_stock_PP = m_stock_PP + m_in_PP - m_out_PP;

m_2 = m_stock;
m_2_PET = m_stock_PET;
m_2_HDPE = m_stock_HDPE; 
m_2_PP = m_stock_PP;

== matlab function NumericalExampleWithSolids/TMN/NODE COMPARTMENT 2 (recycling facility)/Generate impulse14 ==
  data: t input; y output; n_impulse input; mass input
function y = fcn(t, n_impulse, mass)

rectangleWidthToMakeImpulse = 0.4;

y = mass*rectpuls(t-n_impulse,rectangleWidthToMakeImpulse);

== matlab function NumericalExampleWithSolids/TMN/NODE COMPARTMENT 2 (recycling facility)/Generate impulse15 ==
  data: t input; y output; n_impulse input; mass input
function y = fcn(t, n_impulse, mass)

rectangleWidthToMakeImpulse = 0.4;

y = mass*rectpuls(t-n_impulse,rectangleWidthToMakeImpulse);

== matlab function NumericalExampleWithSolids/TMN/NODE COMPARTMENT 2 (recycling facility)/Generate impulse16 ==
  data: t input; y output; n_impulse input; mass input
function y = fcn(t, n_impulse, mass)

rectangleWidthToMakeImpulse = 0.4;

y = mass*rectpuls(t-n_impulse,rectangleWidthToMakeImpulse);

== matlab function NumericalExampleWithSolids/TMN/NODE COMPARTMENT 2 (recycling facility)/Generate impulse17 ==
  data: t input; y output; n_impulse input; mass input
function y = fcn(t, n_impulse, mass)

rectangleWidthToMakeImpulse = 0.4;

y = mass*rectpuls(t-n_impulse,rectangleWidthToMakeImpulse);

== matlab function NumericalExampleWithSolids/TMN/NODE COMPARTMENT 2 (recycling facility)/Generate impulse18 ==
  data: t input; y output; n_impulse input; mass input
function y = fcn(t, n_impulse, mass)

rectangleWidthToMakeImpulse = 0.4;

y = mass*rectpuls(t-n_impulse,rectangleWidthToMakeImpulse);

== matlab function NumericalExampleWithSolids/TMN/NODE COMPARTMENT 1 (organization)/Generate impulse1 ==
  data: t input; y output; n_impulse input; mass input
function y = fcn(t, n_impulse, mass)

rectangleWidthToMakeImpulse = 0.4; % epsilon

y = mass*rectpuls(t-n_impulse,rectangleWidthToMakeImpulse);

== matlab function NumericalExampleWithSolids/TMN/ARC COMPARTMENT 2,1 (transportation)/ARC COMPARTMENT 2_1 ==
  settings: updateMethod=DISCRETE
  data: m_ini_Transport2to1_PET input; m_ini_Transport2to1_HDPE input; m_ini_Transport2to1_PP input; m_in_Transport2to1_PET input; m_in_Transport2to1_HDPE input; m_in_Transport2to1_PP input; m_out_Transport2to1_PET input; m_PET output; m_out_Transport2to1_HDPE input; m_HDPE output; m_PP output; m_out_Transport2to1_PP input
function [m_PET, m_HDPE, m_PP] = fcn(m_ini_Transport2to1_PET, m_ini_Transport2to1_HDPE, m_ini_Transport2to1_PP, m_in_Transport2to1_PET, m_in_Transport2to1_HDPE, m_in_Transport2to1_PP, m_out_Transport2to1_PET, m_out_Transport2to1_HDPE, m_out_Transport2to1_PP)

persistent m_stock_PET;
persistent m_stock_HDPE;
persistent m_stock_PP;

if isempty(m_stock_PET) % t = 0
    m_stock_PET = m_ini_Transport2to1_PET;
    m_stock_HDPE = m_ini_Transport2to1_HDPE; 
    m_stock_PP = m_ini_Transport2to1_PP;
end

m_stock_PET = m_stock_PET + m_in_Transport2to1_PET - m_out_Transport2to1_PET;
m_stock_HDPE = m_stock_HDPE + m_in_Transport2to1_HDPE - m_out_Transport2to1_HDPE;
m_stock_PP = m_stock_PP + m_in_Transport2to1_PP - m_out_Transport2to1_PP;  

m_PET = m_stock_PET;
m_HDPE = m_stock_HDPE;
m_PP = m_stock_PP;

== matlab function NumericalExampleWithSolids/TMN/ARC COMPARTMENT 2,1 (transportation)/Generate impulse19 ==
  data: t input; y output; n_impulse input; mass input
function y = fcn(t, n_impulse, mass)

rectangleWidthToMakeImpulse = 0.4;

y = mass*rectpuls(t-n_impulse,rectangleWidthToMakeImpulse);

== matlab function NumericalExampleWithSolids/TMN/ARC COMPARTMENT 2,1 (transportation)/Generate impulse20 ==
  data: t input; y output; n_impulse input; mass input
function y = fcn(t, n_impulse, mass)

rectangleWidthToMakeImpulse = 0.4;

y = mass*rectpuls(t-n_impulse,rectangleWidthToMakeImpulse);

== matlab function NumericalExampleWithSolids/TMN/ARC COMPARTMENT 2,1 (transportation)/Generate impulse21 ==
  data: t input; y output; n_impulse input; mass input
function y = fcn(t, n_impulse, mass)

rectangleWidthToMakeImpulse = 0.4;

y = mass*rectpuls(t-n_impulse,rectangleWidthToMakeImpulse);

== matlab function NumericalExampleWithSolids/TMN/ARC COMPARTMENT 2,1 (transportation)/Generate impulse22 ==
  data: t input; y output; n_impulse input; mass input
function y = fcn(t, n_impulse, mass)

rectangleWidthToMakeImpulse = 0.4;

y = mass*rectpuls(t-n_impulse,rectangleWidthToMakeImpulse);

== matlab function NumericalExampleWithSolids/TMN/ARC COMPARTMENT 2,1 (transportation)/Generate impulse23 ==
  data: t input; y output; n_impulse input; mass input
function y = fcn(t, n_impulse, mass)

rectangleWidthToMakeImpulse = 0.4;

y = mass*rectpuls(t-n_impulse,rectangleWidthToMakeImpulse);

== matlab function NumericalExampleWithSolids/TMN/ARC COMPARTMENT 2,1 (transportation)/Generate impulse24 ==
  data: t input; y output; n_impulse input; mass input
function y = fcn(t, n_impulse, mass)

rectangleWidthToMakeImpulse = 0.4;

y = mass*rectpuls(t-n_impulse,rectangleWidthToMakeImpulse);

== matlab function NumericalExampleWithSolids/TMN/NODE COMPARTMENT 1 (organization)/Generate impulse25 ==
  data: t input; y output; n_impulse input; mass input
function y = fcn(t, n_impulse, mass)

rectangleWidthToMakeImpulse = 0.4; % epsilon

y = mass*rectpuls(t-n_impulse,rectangleWidthToMakeImpulse);

== matlab function NumericalExampleWithSolids/TMN/NODE COMPARTMENT 1 (organization)/Generate impulse26 ==
  data: t input; y output; n_impulse input; mass input
function y = fcn(t, n_impulse, mass)

rectangleWidthToMakeImpulse = 0.4; % epsilon

y = mass*rectpuls(t-n_impulse,rectangleWidthToMakeImpulse);

== matlab function NumericalExampleWithSolids/TMN/NODE COMPARTMENT 1 (organization)/Generate impulse2 ==
  data: t input; y output; n_impulse input; mass input
function y = fcn(t, n_impulse, mass)

rectangleWidthToMakeImpulse = 0.4; % epsilon

y = mass*rectpuls(t-n_impulse,rectangleWidthToMakeImpulse);

== matlab function NumericalExampleWithSolids/TMN/NODE COMPARTMENT 3 (manufacturer)/NODE COMPARTMENT 3 (manufacturer) ==
  settings: updateMethod=DISCRETE
  data: m_ini_PET input; m_ini_HDPE input; m_ini_PP input; m_3 output; m_out_PET input; m_out_HDPE input; m_out_PP input; m_3_PET output; m_3_HDPE output; m_3_PP output
function [m_3, m_3_PET, m_3_HDPE, m_3_PP] = fcn(m_ini_PET, m_ini_HDPE, m_ini_PP, m_out_PET, m_out_HDPE, m_out_PP)

persistent m_stock;
persistent m_stock_PET;
persistent m_stock_HDPE;
persistent m_stock_PP;

if isempty(m_stock) % t = 0
    m_stock = m_ini_PET + m_ini_HDPE + m_ini_PP;
    m_stock_PET = m_ini_PET;
    m_stock_HDPE = m_ini_HDPE;
    m_stock_PP = m_ini_PP; 
end

m_stock = m_stock - m_out_PET - m_out_HDPE - m_out_PP;
m_stock_PET = m_stock_PET - m_out_PET;
m_stock_HDPE = m_stock_HDPE - m_out_HDPE;
m_stock_PP = m_stock_PP - m_out_PP;

m_3 = m_stock;
m_3_PET = m_stock_PET;
m_3_HDPE = m_stock_HDPE; 
m_3_PP = m_stock_PP;

== matlab function NumericalExampleWithSolids/TMN/NODE COMPARTMENT 3 (manufacturer)/Generate impulse ==
  data: t input; y output; n_impulse input; mass input
function y = fcn(t, n_impulse, mass)

rectangleWidthToMakeImpulse = 0.4; % epsilon

y = mass*rectpuls(t-n_impulse,rectangleWidthToMakeImpulse);

== matlab function NumericalExampleWithSolids/TMN/NODE COMPARTMENT 3 (manufacturer)/Generate impulse1 ==
  data: t input; y output; n_impulse input; mass input
function y = fcn(t, n_impulse, mass)

rectangleWidthToMakeImpulse = 0.4; % epsilon

y = mass*rectpuls(t-n_impulse,rectangleWidthToMakeImpulse);

== matlab function NumericalExampleWithSolids/TMN/NODE COMPARTMENT 3 (manufacturer)/Generate impulse2 ==
  data: t input; y output; n_impulse input; mass input
function y = fcn(t, n_impulse, mass)

rectangleWidthToMakeImpulse = 0.4; % epsilon

y = mass*rectpuls(t-n_impulse,rectangleWidthToMakeImpulse);

== matlab function NumericalExampleWithSolids/TMN/ARC COMPARTMENT 3,1 (transportation)/ARC COMPARTMENT 3_1 ==
  settings: updateMethod=DISCRETE
  data: m_ini_Transport3to1_PET input; m_ini_Transport3to1_HDPE input; m_ini_Transport3to1_PP input; m_in_Transport3to1_PET input; m_in_Transport3to1_HDPE input; m_in_Transport3to1_PP input; m_out_Transport3to1_PET input; m_PET output; m_out_Transport3to1_HDPE input; m_HDPE output; m_PP output; m_out_Transport3to1_PP input
function [m_PET, m_HDPE, m_PP] = fcn(m_ini_Transport3to1_PET, m_ini_Transport3to1_HDPE, m_ini_Transport3to1_PP, m_in_Transport3to1_PET, m_in_Transport3to1_HDPE, m_in_Transport3to1_PP, m_out_Transport3to1_PET, m_out_Transport3to1_HDPE, m_out_Transport3to1_PP)

persistent m_stock_PET;
persistent m_stock_HDPE;
persistent m_stock_PP;

if isempty(m_stock_PET) % t = 0
    m_stock_PET = m_ini_Transport3to1_PET;
    m_stock_HDPE = m_ini_Transport3to1_HDPE; 
    m_stock_PP = m_ini_Transport3to1_PP;
end

m_stock_PET = m_stock_PET + m_in_Transport3to1_PET - m_out_Transport3to1_PET;
m_stock_HDPE = m_stock_HDPE + m_in_Transport3to1_HDPE - m_out_Transport3to1_HDPE;
m_stock_PP = m_stock_PP + m_in_Transport3to1_PP - m_out_Transport3to1_PP;  

m_PET = m_stock_PET;
m_HDPE = m_stock_HDPE;
m_PP = m_stock_PP;

== matlab function NumericalExampleWithSolids/TMN/ARC COMPARTMENT 3,1 (transportation)/Generate impulse19 ==
  data: t input; y output; n_impulse input; mass input
function y = fcn(t, n_impulse, mass)

rectangleWidthToMakeImpulse = 0.4; % epsilon

y = mass*rectpuls(t-n_impulse,rectangleWidthToMakeImpulse);

== matlab function NumericalExampleWithSolids/TMN/ARC COMPARTMENT 3,1 (transportation)/Generate impulse20 ==
  data: t input; y output; n_impulse input; mass input
function y = fcn(t, n_impulse, mass)

rectangleWidthToMakeImpulse = 0.4; % epsilon

y = mass*rectpuls(t-n_impulse,rectangleWidthToMakeImpulse);

== matlab function NumericalExampleWithSolids/TMN/ARC COMPARTMENT 3,1 (transportation)/Generate impulse21 ==
  data: t input; y output; n_impulse input; mass input
function y = fcn(t, n_impulse, mass)

rectangleWidthToMakeImpulse = 0.4; % epsilon

y = mass*rectpuls(t-n_impulse,rectangleWidthToMakeImpulse);

== matlab function NumericalExampleWithSolids/TMN/NODE COMPARTMENT 1 (organization)/NODE COMPARTMENT 1 (organization) ==
  settings: updateMethod=DISCRETE
  data: m_ini_PET input; m_ini_HDPE input; m_ini_PP input; m_in_PET input; m_in_HDPE input; m_in_PP input; m_1 output; m_out_PET input; m_out_HDPE input; m_out_PP input; m_1_PET output; m_1_HDPE output; m_1_PP output
function [m_1, m_1_PET, m_1_HDPE, m_1_PP] = fcn(m_ini_PET, m_ini_HDPE, m_ini_PP, m_in_PET, m_in_HDPE, m_in_PP, m_out_PET, m_out_HDPE, m_out_PP)

persistent m_stock;
persistent m_stock_PET;
persistent m_stock_HDPE;
persistent m_stock_PP;

if isempty(m_stock) % t = 0
    m_stock = m_ini_PET + m_ini_HDPE + m_ini_PP;
    m_stock_PET = m_ini_PET;
    m_stock_HDPE = m_ini_HDPE;
    m_stock_PP = m_ini_PP; 
end

m_stock = m_stock + m_in_PET + m_in_HDPE + m_in_PP - m_out_PET - m_out_HDPE - m_out_PP;
m_stock_PET = m_stock_PET + m_in_PET - m_out_PET;
m_stock_HDPE = m_stock_HDPE + m_in_HDPE - m_out_HDPE;
m_stock_PP = m_stock_PP + m_in_PP - m_out_PP;

m_1 = m_stock;
m_1_PET = m_stock_PET;
m_1_HDPE = m_stock_HDPE; 
m_1_PP = m_stock_PP;

== matlab function NumericalExampleWithSolids/TMN/ARC COMPARTMENT 3,1 (transportation)/Generate impulse22 ==
  data: t input; y output; n_impulse input; mass input
function y = fcn(t, n_impulse, mass)

rectangleWidthToMakeImpulse = 0.4; % epsilon

y = mass*rectpuls(t-n_impulse,rectangleWidthToMakeImpulse);

== matlab function NumericalExampleWithSolids/TMN/ARC COMPARTMENT 3,1 (transportation)/Generate impulse23 ==
  data: t input; y output; n_impulse input; mass input
function y = fcn(t, n_impulse, mass)

rectangleWidthToMakeImpulse = 0.4; % epsilon

y = mass*rectpuls(t-n_impulse,rectangleWidthToMakeImpulse);

== matlab function NumericalExampleWithSolids/TMN/ARC COMPARTMENT 3,1 (transportation)/Generate impulse24 ==
  data: t input; y output; n_impulse input; mass input
function y = fcn(t, n_impulse, mass)

rectangleWidthToMakeImpulse = 0.4; % epsilon

y = mass*rectpuls(t-n_impulse,rectangleWidthToMakeImpulse);

== matlab function NumericalExampleWithSolids/TMN/NODE COMPARTMENT 1 (organization)/Generate impulse ==
  data: t input; y output; n_impulse input; mass input
function y = fcn(t, n_impulse, mass)

rectangleWidthToMakeImpulse = 0.4; % epsilon

y = mass*rectpuls(t-n_impulse,rectangleWidthToMakeImpulse);

== matlab function NumericalExampleWithSolids/TMN/NODE COMPARTMENT 1 (organization)/Generate impulse3 ==
  data: t input; y output; n_impulse input; mass input
function y = fcn(t, n_impulse, mass)

rectangleWidthToMakeImpulse = 0.4; % epsilon

y = mass*rectpuls(t-n_impulse,rectangleWidthToMakeImpulse);

== matlab function NumericalExampleWithSolids/TMN/NODE COMPARTMENT 1 (organization)/Generate impulse4 ==
  data: t input; y output; n_impulse input; mass input
function y = fcn(t, n_impulse, mass)

rectangleWidthToMakeImpulse = 0.4; % epsilon

y = mass*rectpuls(t-n_impulse,rectangleWidthToMakeImpulse);

== matlab function NumericalExampleWithSolids/TMN/NODE COMPARTMENT 1 (organization)/Generate impulse5 ==
  data: t input; y output; n_impulse input; mass input
function y = fcn(t, n_impulse, mass)

rectangleWidthToMakeImpulse = 0.4; % epsilon

y = mass*rectpuls(t-n_impulse,rectangleWidthToMakeImpulse);

== matlab function NumericalExampleWithSolids/TMN/NODE COMPARTMENT 2 (recycling facility)/Generate impulse13 ==
  data: t input; y output; n_impulse input; mass input
function y = fcn(t, n_impulse, mass)

rectangleWidthToMakeImpulse = 0.4;

y = mass*rectpuls(t-n_impulse,rectangleWidthToMakeImpulse);
